simulink model "model"  (R2024b)
settings: Solver=ode1  StartTime=0.0  StopTime=10  FixedStep=0.0001  RelTol=1e-3
values from neighbouring files (symbols this model uses):
  a1 = c*a2    (= 810)    [init.m]
  a2 = c*a3    (= 270)    [init.m]
  a3 = c*a4    (= 90)    [init.m]
  a4 = c*10    (= 30)    [init.m]
  c1 = 50    [init.m]
  c2 = 1    [init.m]
  d = 100    [init.m]
  dis_gain = 30    [init.m]
  epsilon = 1    [init.m]
  i = 20    [init.m]
  k = 5    [init.m]
  mu = 0.9    [init.m]
  p = 400    [init.m]
  phi_frist = 0    [init.m]
  psi_frist = 0    [init.m]
  tau_p_max = 3000000    [init.m]
  theta_frist = 0    [init.m]
  umax = pi/2 - 0.01    (= 1.56079632679)    [init.m]
  w = wo    (= 50)    [init.m]
  wo = 50    [init.m]
  x_frist = 0    [init.m]
  y_frist = 0    [init.m]
  z_frist = 0    [init.m]
libraries: fod x36, slpidlib x6, simulink x1
(part 1 of 4)
settings Model: Creator=qians  LastModifiedBy=qians

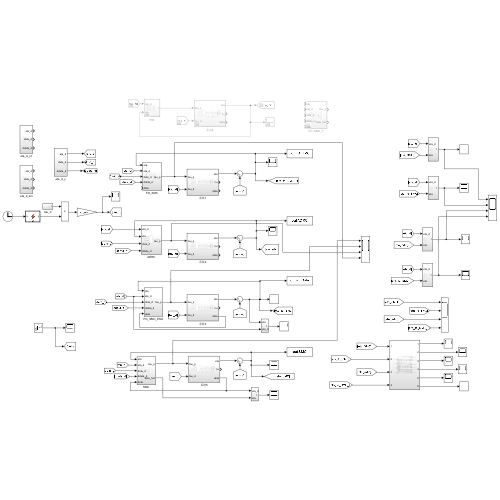
[thumbnail: Simulink's stored preview of the top-level diagram]
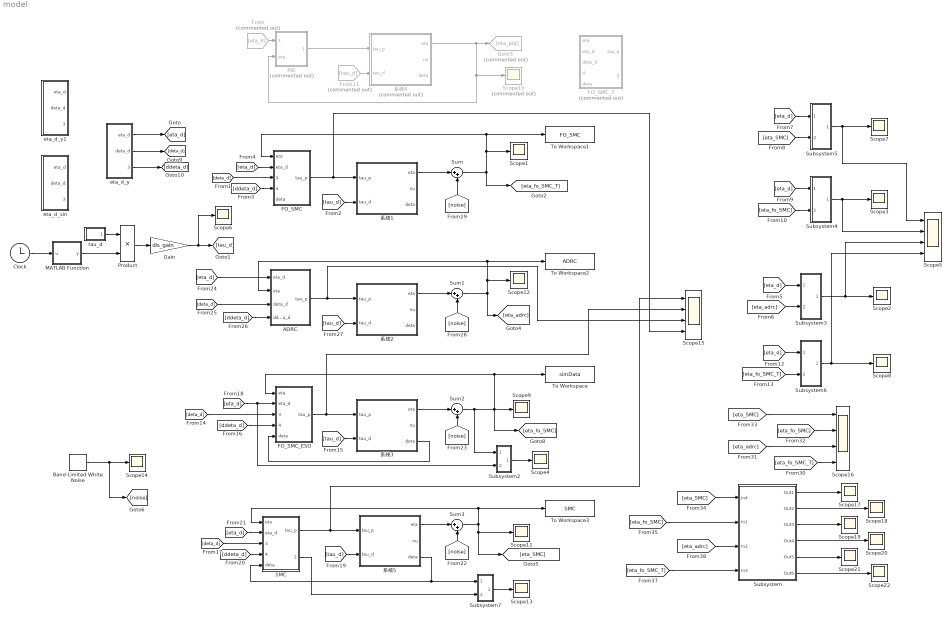
== system model ==
  ADRC : Subsystem
  Band-Limited White Noise : simulink/Sources/Band-Limited White Noise  Cov=[0.00001]  Ts=0.001  seed=[23341]
  Clock : Clock
  FO_SMC : Subsystem
  FO_SMC_ESO : Subsystem
  FO_SMC_T : Subsystem  Commented=on
  From : From  Commented=on  GotoTag=eta_d
  From11 : From  Commented=on  GotoTag=tau_d
  Gain : Gain  Gain=dis_gain
  Goto3 : Goto  Commented=on  GotoTag=eta_pid
  MATLAB Function : MATLAB Function  TreatAsAtomicUnit=on
  PID : Subsystem  Commented=on
  Product : Product
  SMC : Subsystem
  Scope{1..4,6..9,11..14,17..22} (18 alike) : Scope
  Scope10 : Scope  Commented=on
  Scope15 : Scope  NumInputPorts=4
  Scope16 : Scope  NumInputPorts=4
  Scope5 : Scope  NumInputPorts=4
  Subsystem : Subsystem
  Subsystem2 : Subsystem
  Subsystem3 : Subsystem
  Subsystem4 : Subsystem
  Subsystem5 : Subsystem
  Subsystem6 : Subsystem
  Subsystem7 : Subsystem
  Sum{,1..3} (4 alike) : Sum  Inputs=|++
  To Workspace : ToWorkspace  VariableName=simData  SaveFormat=Structure With Time  SampleTime=-1
  To Workspace1 : ToWorkspace  VariableName=FO_SMC  SaveFormat=Structure With Time  SampleTime=-1
  To Workspace2 : ToWorkspace  VariableName=ADRC  SaveFormat=Structure With Time  SampleTime=-1
  To Workspace3 : ToWorkspace  VariableName=SMC  SaveFormat=Structure With Time  SampleTime=-1
  eta_d_sin : Subsystem
  eta_d_y : Subsystem
  eta_d_y1 : Subsystem
  tau_d : Subsystem
  系统1 : Subsystem
  系统2 : Subsystem
  系统3 : Subsystem
  系统4 : Subsystem  Commented=on
  系统5 : Subsystem
  wires:
  Sum2/1 -> Subsystem2/1(eta), FO_SMC_ESO/1(eta), To Workspace/1, Scope9/1, [eta_fo_SMC]
  eta_d_y/2(deta_d) -> [deta_d]
  eta_d_y/1(eta_d) -> [eta_d]
  [deta_d] -> FO_SMC_ESO/3(deta_d)
  [ddeta_d] -> FO_SMC_ESO/4(ddeta_d)
  系统3/3(deta) -> FO_SMC_ESO/5(deta)
  [eta_d] -> FO_SMC_ESO/2(eta_d), Subsystem2/2(eta_d)
  eta_d_y/3(ddeta_d) -> [ddeta_d]
  FO_SMC_ESO/1(tau_p) -> 系统3/1(tau_p), Scope15/2
  [tau_d] -> 系统3/2(tau_d)
  Subsystem2/1(Out1) -> Scope4/1
  [ddeta_d] -> FO_SMC/4(ddeta_d)
  [tau_d] -> 系统1/2(tau_d)
  FO_SMC/1(tau_p) -> 系统1/1(tau_p), Scope15/4
  [eta_d] -> FO_SMC/2(eta_d)
  Sum/1 -> To Workspace1/1, FO_SMC/1(eta), Scope1/1, [eta_fo_SMC_T]
  [deta_d] -> FO_SMC/3(deta_d)
  [eta_SMC] -> Subsystem5/2(eta)
  [eta_fo_SMC_T] -> Subsystem6/2(eta)
  [eta_d] -> Subsystem3/1(eta_d)
  [eta_adrc] -> Subsystem3/2(eta)
  [eta_d] -> Subsystem5/1(eta_d)
  [eta_d] -> Subsystem4/1(eta_d)
  Subsystem3/1(Out1) -> Scope5/3, Scope2/1
  Subsystem5/1(Out1) -> Scope5/1, Scope7/1
  [eta_d] -> Subsystem6/1(eta_d)
  [eta_fo_SMC] -> Subsystem4/2(eta)
  Subsystem6/1(Out1) -> Scope5/4, Scope8/1
  Subsystem4/1(Out1) -> Scope5/2, Scope3/1
  From11/1 -> 系统4/2(tau_d)
  From/1 -> PID/1(eta_d)
  PID/1(Out1) -> 系统4/1(tau_p)
  系统4/1(eta) -> Scope10/1, PID/2(eta), Goto3/1
  [ddeta_d] -> ADRC/4(ddeta_d)
  ADRC/1(tau_p) -> Scope15/3, 系统2/1(tau_p)
  [tau_d] -> 系统2/2(tau_d)
  Sum1/1 -> ADRC/2(eta), To Workspace2/1, Scope12/1, [eta_adrc]
  [deta_d] -> ADRC/3(deta_d)
  [eta_d] -> ADRC/1(eta_d)
  [ddeta_d] -> SMC/4(ddeta_d)
  [deta_d] -> SMC/3(deta_d)
  [eta_d] -> SMC/2(eta_d)
  SMC/1(tau_p) -> 系统5/1(tau_p), Scope15/1
  Sum3/1 -> Scope11/1, [eta_SMC], SMC/1(eta), To Workspace3/1
  系统5/3(deta) -> SMC/5(deta), Subsystem7/1(eta_d)
  Subsystem7/1(Out1) -> Scope13/1
  [tau_d] -> 系统5/2(tau_d)
  SMC/2(deta_hat) -> Subsystem7/2(eta)
  Gain/1 -> [tau_d], Scope6/1
  Band-Limited White Noise/1 -> [noise], Scope14/1
  系统1/1(eta) -> Sum/1
  系统2/1(eta) -> Sum1/1
  系统3/1(eta) -> Sum2/1
  系统5/1(eta) -> Sum3/1
  [noise] -> Sum1/2
  [noise] -> Sum/2
  tau_d/1(Out1) -> Product/1
  Product/1 -> Gain/1
  Clock/1 -> MATLAB Function/1(u)
  MATLAB Function/1(y) -> Product/2
  [eta_fo_SMC_T] -> Scope16/4
  [eta_adrc] -> Scope16/3
  [eta_fo_SMC] -> Scope16/2
  [eta_SMC] -> Scope16/1
  [eta_SMC] -> Subsystem/1(In4)
  [eta_fo_SMC] -> Subsystem/2(In1)
  [eta_adrc] -> Subsystem/3(In2)
  [eta_fo_SMC_T] -> Subsystem/4(In3)
  Subsystem/1(Out1) -> Scope17/1
  Subsystem/2(Out2) -> Scope18/1
  Subsystem/3(Out3) -> Scope19/1
  Subsystem/4(Out4) -> Scope20/1
  Subsystem/5(Out5) -> Scope21/1
  Subsystem/6(Out6) -> Scope22/1
  [noise] -> Sum2/2
  [noise] -> Sum3/2

== system model/ADRC ==
  eta_d : Inport
  eta : Inport  Port=2
  deta_d : Inport  Port=3
  ddeta_d : Inport  Port=4
  控制器 : Subsystem
  tau_p : Outport
  wires:
  ddeta_d/1 -> 控制器/4(ddr)
  deta_d/1 -> 控制器/3(dr)
  eta/1 -> 控制器/2(eta)
  eta_d/1 -> 控制器/1(r)
  控制器/1(tau_p) -> tau_p/1

== system model/FO_SMC ==
  eta : Inport
  eta_d : Inport  Port=2
  deta_d : Inport  Port=3
  ddeta_d : Inport  Port=4
  deta : Inport  Port=5
  Constant : Constant  Value=c1
  Constant1 : Constant  Value=c2
  Constant2 : Constant  Value=k
  Constant3 : Constant  Value=epsilon
  MATLAB Function : MATLAB Function  TreatAsAtomicUnit=on
  MATLAB Function1 : MATLAB Function  TreatAsAtomicUnit=on
  Subsystem : Subsystem
  Subsystem2 : Subsystem
  tau_p : Outport
  wires:
  MATLAB Function1/1(nu) -> MATLAB Function/6(nu)
  eta_d/1 -> Subsystem2/2(eta_d), MATLAB Function/2(eta_d)
  ddeta_d/1 -> MATLAB Function/5(ddeta_d)
  eta/1 -> Subsystem/1(y), MATLAB Function1/1(eta), Subsystem2/1(eta), MATLAB Function/1(eta)
  Subsystem2/1(Out1) -> MATLAB Function/7(D1)
  Subsystem2/2(Out2) -> MATLAB Function/8(D2)
  deta_d/1 -> MATLAB Function/4(deta_d)
  Subsystem/2(y1_hat) -> MATLAB Function/3(deta), MATLAB Function1/2(deta)
  Constant/1 -> MATLAB Function/9(c1)
  Constant1/1 -> MATLAB Function/10(c2)
  Constant2/1 -> MATLAB Function/11(k)
  Constant3/1 -> MATLAB Function/12(epsilon)
  MATLAB Function/1(tau_p) -> tau_p/1

== system model/FO_SMC_ESO ==
  eta : Inport
  eta_d : Inport  Port=2
  deta_d : Inport  Port=3
  ddeta_d : Inport  Port=4
  deta : Inport  Port=5
  LESO : Subsystem
  Levant微分器 : Subsystem
  MATLAB Function : MATLAB Function  TreatAsAtomicUnit=on
  Subsystem1 : Subsystem
  Subsystem2 : Subsystem
  Subsystem3 : Subsystem
  Sum1 : Sum  Inputs=|++
  tau_p : Outport
  wires:
  Sum1/1 -> MATLAB Function/2(u2), LESO/5(tau_c)
  LESO/1(tau_2) -> Sum1/1
  eta/1 -> Subsystem3/1(eta), Subsystem2/1(eta), LESO/1(eta), Levant微分器/1(y), Subsystem2/3(eta1), Subsystem3/2(eta1)
  Levant微分器/2(y1_hat) -> Subsystem2/2(deta), Subsystem3/5(deta), Subsystem2/4(deta1)
  Subsystem1/1(Out1) -> tau_p/1
  MATLAB Function/1(y) -> Subsystem1/1(y)
  Subsystem3/1(tau_3) -> Sum1/2
  eta_d/1 -> Subsystem3/6(eta_d)
  deta_d/1 -> Subsystem3/7(deta_d)
  ddeta_d/1 -> Subsystem3/8(ddeta_d)
  Subsystem2/3(J) -> Subsystem3/4(J), LESO/3(J)
  Subsystem2/2(M_eta) -> Subsystem3/3(M_eta), LESO/2(M_eta)
  Subsystem2/1(tau_1) -> MATLAB Function/1(u1)
  Subsystem2/4(J_inv) -> LESO/4(J_inv)
  LESO/2(h3) -> Subsystem3/9(h3)

== system model/FO_SMC_T ==
  eta : Inport
  eta_d : Inport  Port=2
  deta_d : Inport  Port=3
  ddeta_d : Inport  Port=4
  deta : Inport  Port=5
  Constant1 : Constant  Value=c1
  Constant2 : Constant  Value=k
  Constant3 : Constant  Value=epsilon
  Constant4 : Constant  Value=c2
  MATLAB Function : MATLAB Function  TreatAsAtomicUnit=on
  MATLAB Function1 : MATLAB Function  TreatAsAtomicUnit=on
  Subsystem : Subsystem
  Subsystem2 : Subsystem
  tau_p : Outport
  deta_hat : Outport  Port=2
  wires:
  MATLAB Function/1(tau_p) -> tau_p/1
  MATLAB Function1/1(nu) -> MATLAB Function/6(nu)
  eta_d/1 -> Subsystem2/2(eta_d), MATLAB Function/2(eta_d)
  ddeta_d/1 -> MATLAB Function/5(ddeta_d)
  Subsystem2/1(Out1) -> MATLAB Function/7(D1)
  Subsystem2/2(Out2) -> MATLAB Function/8(D2)
  deta_d/1 -> MATLAB Function/4(deta_d)
  Subsystem/2(y1_hat) -> MATLAB Function/3(deta), MATLAB Function1/2(deta), deta_hat/1
  eta/1 -> Subsystem/1(y), Subsystem2/1(eta), MATLAB Function1/1(eta)
  Subsystem/1(y_hat) -> MATLAB Function/1(eta)
  Constant2/1 -> MATLAB Function/9(k)
  Constant3/1 -> MATLAB Function/10(epsilon)
  Constant1/1 -> MATLAB Function/11(c1)
  Constant4/1 -> MATLAB Function/12(c2)

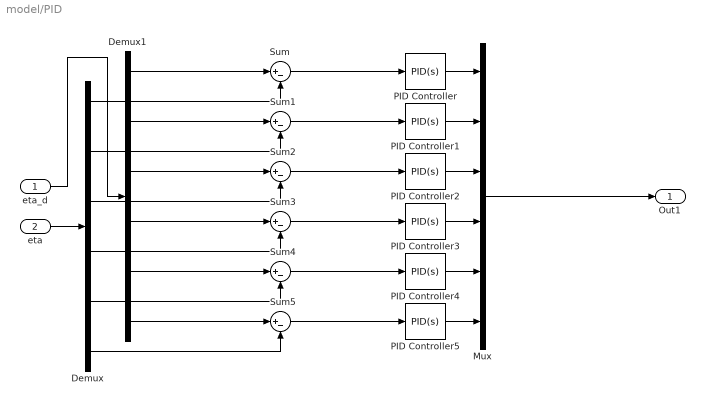
== system model/PID ==
  eta_d : Inport
  eta : Inport  Port=2
  Demux : Demux  Outputs=6
  Demux1 : Demux  Outputs=6
  Mux : Mux  Inputs=6
  PID Controller{,1..5} (6 alike) : slpidlib/PID Controller  Controller=PID  Form=Parallel  TimeDomain=Continuous-time  UseExternalTs=off  SampleTime=-1  IntegratorMethod=Forward Euler  FilterMethod=Forward Euler  ControllerParametersSource=internal  P=p  I=i  UseKiTs=off  D=d  UseExternalDerivativeSource=off  N=100  UseFilter=on  TunerSelectOption=Transfer Function Based (PID Tuner App)  InitialConditionSource=internal  InitialConditionForIntegrator=0  InitialConditionForFilter=0  DifferentiatorICPrevScaledInput=0  ExternalReset=none  TrackingMode=off  Kt=1  LimitOutput=off  SatLimitsSource=internal  UpperSaturationLimit=inf  LowerSaturationLimit=-inf  LinearizeAsGain=on  AntiWindupMode=none  Kb=1  LimitIntegrator=off  UpperIntegratorSaturationLimit=inf  LowerIntegratorSaturationLimit=-inf  POutMin=[]  POutMax=[]  IOutMin=[]  IOutMax=[]  DOutMin=[]  DOutMax=[]  NOutMin=[]  NOutMax=[]  SumOutMin=[]  SumOutMax=[]  SaturationOutMin=[]  SaturationOutMax=[]  PParamMin=[]  PParamMax=[]  IParamMin=[]  IParamMax=[]  DParamMin=[]  DParamMax=[]  NParamMin=[]  NParamMax=[]  KbParamMin=[]  KbParamMax=[]  KtParamMin=[]  KtParamMax=[]  KbOutMin=[]  KbOutMax=[]  KtOutMin=[]  KtOutMax=[]  IntegratorOutMin=[]  IntegratorOutMax=[]  FilterOutMin=[]  FilterOutMax=[]  SumI1OutMin=[]  SumI1OutMax=[]  SumI2OutMin=[]  SumI2OutMax=[]  SumI3OutMin=[]  SumI3OutMax=[]  SumI4OutMin=[]  SumI4OutMax=[]  SumDOutMin=[]  SumDOutMax=[]  DifferentiatorOutMin=[]  DifferentiatorOutMax=[]  FilterDiffOutCoefMin=[]  FilterDiffOutCoefMax=[]  ReciprocalOutMin=[]  ReciprocalOutMax=[]  SumDenOutMin=[]  SumDenOutMax=[]  SumNumOutMin=[]  SumNumOutMax=[]  DivideOutMin=[]  DivideOutMax=[]  UdiffTsProdOutMin=[]  UdiffTsProdOutMax=[]  NTsProdOutMin=[]  NTsProdOutMax=[]  UintegralTsProdOutMin=[]  UintegralTsProdOutMax=[]  UngainTsProdOutMin=[]  UngainTsProdOutMax=[]  ClampingZeroOutDataTypeStr=Inherit: Inherit via back propagation  ClampingZeroOutMin=[]  ClampingZeroOutMax=[]  FilterDenConstantOutDataTypeStr=Inherit: Inherit via back propagation  FilterDenConstantOutMin=[]  FilterDenConstantOutMax=[]  PCopyOutDataTypeStr=Inherit: Inherit via back propagation  PCopyOutMin=[]  PCopyOutMax=[]  NCopyOutDataTypeStr=Inherit: Inherit via back propagation  NCopyOutMin=[]  NCopyOutMax=[]  IntegratorContinuousStateAttributes=''  IntegratorStateMustResolveToSignalObject=off  IntegratorRTWStateStorageClass=Auto  FilterContinuousStateAttributes=''  FilterStateMustResolveToSignalObject=off  FilterRTWStateStorageClass=Auto  ParallelPVariant=InternalParameters  IdealPVariant=Disabled  IVariant=InternalParameters  DVariant=InternalParameters  IntegratorVariant=Continuous  SatVariant=Disabled  AWVariant=Passthrough  PCopyVariant=Disabled  TRVariant=Disabled  FdbkBlocksVariant=Forward  IdealPFdbkVariant=Disabled  SatFdbkVariant=Disabled  DerivativeFilterVariant=ContFilter  NVariant=InternalParameters  NCopyVariant=Disabled  FilterICVariant=InternalICsFilter  IntegratorICVariant=InternalICs  ExternalResetVariant=Disabled  TRSumVariant=Passthrough  SumFdbkVariant=Disabled  SumVariant=Sum_PID  TsampFilterVariant=InternalTs  TsampNgainVariant=Passthrough  TsampIntegralVariant=Disabled_SignalSpec  ExternalSaturationOutDataTypeStr=Inherit: Same as second input  DerivativeSourceVariant=ErrorSignal  PreIntVariant=InternalPreInt
  Sum{,1..5} (6 alike) : Sum  Inputs=|+-
  Out1 : Outport
  wires:
  PID Controller5/1 -> Mux/6
  PID Controller/1 -> Mux/1
  PID Controller4/1 -> Mux/5
  PID Controller2/1 -> Mux/3
  PID Controller1/1 -> Mux/2
  PID Controller3/1 -> Mux/4
  Mux/1 -> Out1/1
  eta/1 -> Demux/1
  Demux1/1 -> Sum/1
  Sum/1 -> PID Controller/1
  Demux/1 -> Sum/2
  Demux/2 -> Sum1/2
  Sum1/1 -> PID Controller1/1
  Demux1/2 -> Sum1/1
  Demux1/3 -> Sum2/1
  Sum2/1 -> PID Controller2/1
  Demux/3 -> Sum2/2
  Demux/4 -> Sum3/2
  Sum3/1 -> PID Controller3/1
  Demux1/4 -> Sum3/1
  Demux1/5 -> Sum4/1
  Sum4/1 -> PID Controller4/1
  Demux/5 -> Sum4/2
  Demux/6 -> Sum5/2
  Sum5/1 -> PID Controller5/1
  Demux1/6 -> Sum5/1
  eta_d/1 -> Demux1/1

== system model/SMC ==
  eta : Inport
  eta_d : Inport  Port=2
  deta_d : Inport  Port=3
  ddeta_d : Inport  Port=4
  deta : Inport  Port=5
  Constant : Constant  Value=c1
  Constant2 : Constant  Value=k
  Constant3 : Constant  Value=epsilon
  MATLAB Function : MATLAB Function  TreatAsAtomicUnit=on
  MATLAB Function1 : MATLAB Function  TreatAsAtomicUnit=on
  Subsystem : Subsystem
  tau_p : Outport
  deta_hat : Outport  Port=2
  wires:
  MATLAB Function/1(tau_p) -> tau_p/1
  MATLAB Function1/1(nu) -> MATLAB Function/6(nu)
  eta_d/1 -> MATLAB Function/2(eta_d)
  ddeta_d/1 -> MATLAB Function/5(ddeta_d)
  eta/1 -> MATLAB Function/1(eta), MATLAB Function1/1(eta), Subsystem/1(y)
  deta_d/1 -> MATLAB Function/4(deta_d)
  Subsystem/2(y1_hat) -> deta_hat/1, MATLAB Function/3(deta), MATLAB Function1/2(deta)
  Constant/1 -> MATLAB Function/7(c1)
  Constant2/1 -> MATLAB Function/8(k)
  Constant3/1 -> MATLAB Function/9(epsilon)

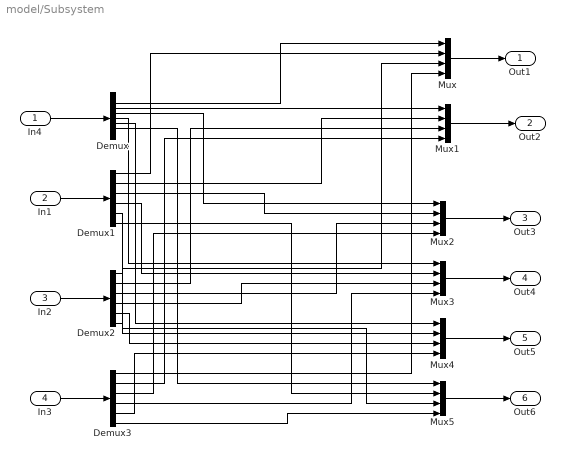
== system model/Subsystem ==
  In4 : Inport
  In1 : Inport  Port=2
  In2 : Inport  Port=3
  In3 : Inport  Port=4
  Demux{,1..3} (4 alike) : Demux  Outputs=6
  Mux{,1..5} (6 alike) : Mux
  Out1 : Outport
  Out2 : Outport  Port=2
  Out3 : Outport  Port=3
  Out4 : Outport  Port=4
  Out5 : Outport  Port=5
  Out6 : Outport  Port=6
  wires:
  Demux/1 -> Mux/1
  In4/1 -> Demux/1
  Mux/1 -> Out1/1
  In1/1 -> Demux1/1
  Demux1/1 -> Mux/2
  Demux/2 -> Mux1/1
  Demux1/2 -> Mux1/2
  Mux1/1 -> Out2/1
  Mux2/1 -> Out3/1
  Demux1/3 -> Mux2/2
  Demux/3 -> Mux2/1
  Demux/4 -> Mux3/1
  Demux1/4 -> Mux3/2
  Mux3/1 -> Out4/1
  Mux4/1 -> Out5/1
  Demux1/5 -> Mux4/2
  Demux/5 -> Mux4/1
  Demux/6 -> Mux5/1
  Demux1/6 -> Mux5/2
  Mux5/1 -> Out6/1
  In2/1 -> Demux2/1
  In3/1 -> Demux3/1
  Demux2/1 -> Mux/3
  Demux2/2 -> Mux1/3
  Demux2/3 -> Mux2/3
  Demux2/4 -> Mux3/3
  Demux2/5 -> Mux4/3
  Demux2/6 -> Mux5/3
  Demux3/1 -> Mux/4
  Demux3/2 -> Mux1/4
  Demux3/3 -> Mux2/4
  Demux3/4 -> Mux3/4
  Demux3/5 -> Mux4/4
  Demux3/6 -> Mux5/4

== system model/Subsystem2 ==
  eta : Inport
  eta_d : Inport  Port=2
  Demux : Demux  Outputs=6
  Demux1 : Demux  Outputs=6
  Mux : Mux  Inputs=6
  Sum{,1..5} (6 alike) : Sum  Inputs=|+-
  Out1 : Outport
  wires:
  eta_d/1 -> Demux1/1
  Demux1/6 -> Sum5/1
  Demux/6 -> Sum5/2
  Demux/5 -> Sum4/2
  Demux1/5 -> Sum4/1
  Demux1/4 -> Sum3/1
  Demux/4 -> Sum3/2
  Demux/3 -> Sum2/2
  Demux1/3 -> Sum2/1
  Demux1/2 -> Sum1/1
  Demux/2 -> Sum1/2
  Demux/1 -> Sum/2
  Demux1/1 -> Sum/1
  eta/1 -> Demux/1
  Mux/1 -> Out1/1
  Sum3/1 -> Mux/4
  Sum1/1 -> Mux/2
  Sum2/1 -> Mux/3
  Sum4/1 -> Mux/5
  Sum/1 -> Mux/1
  Sum5/1 -> Mux/6

== system model/Subsystem3 ==
  eta_d : Inport
  eta : Inport  Port=2
  Demux : Demux  Outputs=6
  Demux1 : Demux  Outputs=6
  Mux : Mux  Inputs=6
  Sum{,1..5} (6 alike) : Sum  Inputs=|+-
  Out1 : Outport
  wires:
  eta_d/1 -> Demux1/1
  Demux1/6 -> Sum5/1
  Demux/6 -> Sum5/2
  Demux/5 -> Sum4/2
  Demux1/5 -> Sum4/1
  Demux1/4 -> Sum3/1
  Demux/4 -> Sum3/2
  Demux/3 -> Sum2/2
  Demux1/3 -> Sum2/1
  Demux1/2 -> Sum1/1
  Demux/2 -> Sum1/2
  Demux/1 -> Sum/2
  Demux1/1 -> Sum/1
  eta/1 -> Demux/1
  Mux/1 -> Out1/1
  Sum3/1 -> Mux/4
  Sum1/1 -> Mux/2
  Sum2/1 -> Mux/3
  Sum4/1 -> Mux/5
  Sum/1 -> Mux/1
  Sum5/1 -> Mux/6

== system model/Subsystem4 ==
  eta_d : Inport
  eta : Inport  Port=2
  Demux : Demux  Outputs=6
  Demux1 : Demux  Outputs=6
  Mux : Mux  Inputs=6
  Sum{,1..5} (6 alike) : Sum  Inputs=|+-
  Out1 : Outport
  wires:
  Sum5/1 -> Mux/6
  Sum/1 -> Mux/1
  Sum4/1 -> Mux/5
  Sum2/1 -> Mux/3
  Sum1/1 -> Mux/2
  Sum3/1 -> Mux/4
  Mux/1 -> Out1/1
  eta/1 -> Demux/1
  Demux1/1 -> Sum/1
  Demux/1 -> Sum/2
  Demux/2 -> Sum1/2
  Demux1/2 -> Sum1/1
  Demux1/3 -> Sum2/1
  Demux/3 -> Sum2/2
  Demux/4 -> Sum3/2
  Demux1/4 -> Sum3/1
  Demux1/5 -> Sum4/1
  Demux/5 -> Sum4/2
  Demux/6 -> Sum5/2
  Demux1/6 -> Sum5/1
  eta_d/1 -> Demux1/1

== system model/Subsystem5 ==
  eta_d : Inport
  eta : Inport  Port=2
  Demux : Demux  Outputs=6
  Demux1 : Demux  Outputs=6
  Mux : Mux  Inputs=6
  Sum{,1..5} (6 alike) : Sum  Inputs=|+-
  Out1 : Outport
  wires:
  eta_d/1 -> Demux1/1
  Demux1/6 -> Sum5/1
  Demux/6 -> Sum5/2
  Demux/5 -> Sum4/2
  Demux1/5 -> Sum4/1
  Demux1/4 -> Sum3/1
  Demux/4 -> Sum3/2
  Demux/3 -> Sum2/2
  Demux1/3 -> Sum2/1
  Demux1/2 -> Sum1/1
  Demux/2 -> Sum1/2
  Demux/1 -> Sum/2
  Demux1/1 -> Sum/1
  eta/1 -> Demux/1
  Mux/1 -> Out1/1
  Sum3/1 -> Mux/4
  Sum1/1 -> Mux/2
  Sum2/1 -> Mux/3
  Sum4/1 -> Mux/5
  Sum/1 -> Mux/1
  Sum5/1 -> Mux/6

== system model/Subsystem6 ==
  eta_d : Inport
  eta : Inport  Port=2
  Demux : Demux  Outputs=6
  Demux1 : Demux  Outputs=6
  Mux : Mux  Inputs=6
  Sum{,1..5} (6 alike) : Sum  Inputs=|+-
  Out1 : Outport
  wires:
  Sum5/1 -> Mux/6
  Sum/1 -> Mux/1
  Sum4/1 -> Mux/5
  Sum2/1 -> Mux/3
  Sum1/1 -> Mux/2
  Sum3/1 -> Mux/4
  Mux/1 -> Out1/1
  eta/1 -> Demux/1
  Demux1/1 -> Sum/1
  Demux/1 -> Sum/2
  Demux/2 -> Sum1/2
  Demux1/2 -> Sum1/1
  Demux1/3 -> Sum2/1
  Demux/3 -> Sum2/2
  Demux/4 -> Sum3/2
  Demux1/4 -> Sum3/1
  Demux1/5 -> Sum4/1
  Demux/5 -> Sum4/2
  Demux/6 -> Sum5/2
  Demux1/6 -> Sum5/1
  eta_d/1 -> Demux1/1

== system model/Subsystem7 ==
  eta_d : Inport
  eta : Inport  Port=2
  Demux : Demux  Outputs=6
  Demux1 : Demux  Outputs=6
  Mux : Mux  Inputs=6
  Sum{,1..5} (6 alike) : Sum  Inputs=|+-
  Out1 : Outport
  wires:
  eta_d/1 -> Demux1/1
  Demux1/6 -> Sum5/1
  Demux/6 -> Sum5/2
  Demux/5 -> Sum4/2
  Demux1/5 -> Sum4/1
  Demux1/4 -> Sum3/1
  Demux/4 -> Sum3/2
  Demux/3 -> Sum2/2
  Demux1/3 -> Sum2/1
  Demux1/2 -> Sum1/1
  Demux/2 -> Sum1/2
  Demux/1 -> Sum/2
  Demux1/1 -> Sum/1
  eta/1 -> Demux/1
  Mux/1 -> Out1/1
  Sum3/1 -> Mux/4
  Sum1/1 -> Mux/2
  Sum2/1 -> Mux/3
  Sum4/1 -> Mux/5
  Sum/1 -> Mux/1
  Sum5/1 -> Mux/6

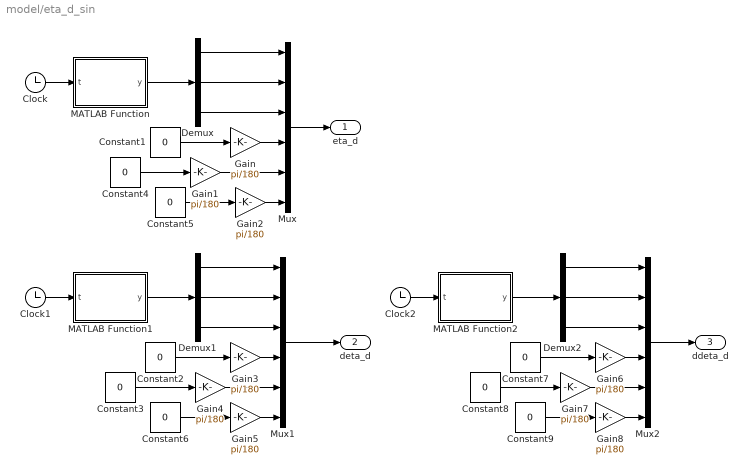
== system model/eta_d_sin ==
  Clock : Clock
  Clock1 : Clock
  Clock2 : Clock
  Constant{1..9} (9 alike) : Constant  Value=0
  Demux : Demux  Outputs=3
  Demux1 : Demux  Outputs=3
  Demux2 : Demux  Outputs=3
  Gain{,1..8} (9 alike) : Gain  Gain=pi/180
  MATLAB Function : MATLAB Function  TreatAsAtomicUnit=on
  MATLAB Function1 : MATLAB Function  TreatAsAtomicUnit=on
  MATLAB Function2 : MATLAB Function  TreatAsAtomicUnit=on
  Mux : Mux  Inputs=6
  Mux1 : Mux  Inputs=6
  Mux2 : Mux  Inputs=6
  eta_d : Outport
  deta_d : Outport  Port=2
  ddeta_d : Outport  Port=3
  wires:
  Gain2/1 -> Mux/6
  Demux/1 -> Mux/1
  Gain/1 -> Mux/4
  Constant4/1 -> Gain1/1
  Mux/1 -> eta_d/1
  Demux/3 -> Mux/3
  Demux/2 -> Mux/2
  Constant5/1 -> Gain2/1
  Gain1/1 -> Mux/5
  Constant1/1 -> Gain/1
  Clock/1 -> MATLAB Function/1(t)
  MATLAB Function/1(y) -> Demux/1
  MATLAB Function1/1(y) -> Demux1/1
  Clock1/1 -> MATLAB Function1/1(t)
  Constant2/1 -> Gain3/1
  Gain4/1 -> Mux1/5
  Constant6/1 -> Gain5/1
  Demux1/2 -> Mux1/2
  Demux1/3 -> Mux1/3
  Mux1/1 -> deta_d/1
  Constant3/1 -> Gain4/1
  Gain3/1 -> Mux1/4
  Demux1/1 -> Mux1/1
  Gain5/1 -> Mux1/6
  Gain8/1 -> Mux2/6
  Demux2/1 -> Mux2/1
  Gain6/1 -> Mux2/4
  Constant8/1 -> Gain7/1
  Mux2/1 -> ddeta_d/1
  Demux2/3 -> Mux2/3
  Demux2/2 -> Mux2/2
  Constant9/1 -> Gain8/1
  Gain7/1 -> Mux2/5
  Constant7/1 -> Gain6/1
  Clock2/1 -> MATLAB Function2/1(t)
  MATLAB Function2/1(y) -> Demux2/1

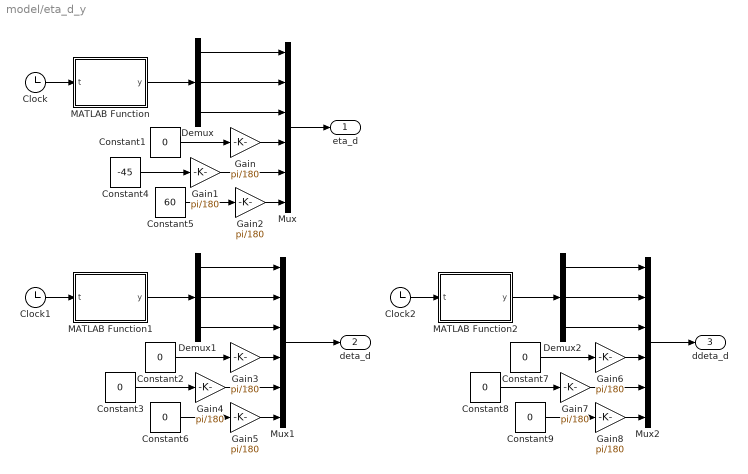
== system model/eta_d_y ==
  Clock : Clock
  Clock1 : Clock
  Clock2 : Clock
  Constant{1..3,6..9} (7 alike) : Constant  Value=0
  Constant4 : Constant  Value=-45
  Constant5 : Constant  Value=60
  Demux : Demux  Outputs=3
  Demux1 : Demux  Outputs=3
  Demux2 : Demux  Outputs=3
  Gain{,1..8} (9 alike) : Gain  Gain=pi/180
  MATLAB Function : MATLAB Function  TreatAsAtomicUnit=on
  MATLAB Function1 : MATLAB Function  TreatAsAtomicUnit=on
  MATLAB Function2 : MATLAB Function  TreatAsAtomicUnit=on
  Mux : Mux  Inputs=6
  Mux1 : Mux  Inputs=6
  Mux2 : Mux  Inputs=6
  eta_d : Outport
  deta_d : Outport  Port=2
  ddeta_d : Outport  Port=3
  wires:
  Gain2/1 -> Mux/6
  Demux/1 -> Mux/1
  Gain/1 -> Mux/4
  Constant4/1 -> Gain1/1
  Mux/1 -> eta_d/1
  Demux/3 -> Mux/3
  Demux/2 -> Mux/2
  Constant5/1 -> Gain2/1
  Gain1/1 -> Mux/5
  Constant1/1 -> Gain/1
  Clock/1 -> MATLAB Function/1(t)
  MATLAB Function/1(y) -> Demux/1
  MATLAB Function1/1(y) -> Demux1/1
  Clock1/1 -> MATLAB Function1/1(t)
  Constant2/1 -> Gain3/1
  Gain4/1 -> Mux1/5
  Constant6/1 -> Gain5/1
  Demux1/2 -> Mux1/2
  Demux1/3 -> Mux1/3
  Mux1/1 -> deta_d/1
  Constant3/1 -> Gain4/1
  Gain3/1 -> Mux1/4
  Demux1/1 -> Mux1/1
  Gain5/1 -> Mux1/6
  Gain8/1 -> Mux2/6
  Demux2/1 -> Mux2/1
  Gain6/1 -> Mux2/4
  Constant8/1 -> Gain7/1
  Mux2/1 -> ddeta_d/1
  Demux2/3 -> Mux2/3
  Demux2/2 -> Mux2/2
  Constant9/1 -> Gain8/1
  Gain7/1 -> Mux2/5
  Constant7/1 -> Gain6/1
  Clock2/1 -> MATLAB Function2/1(t)
  MATLAB Function2/1(y) -> Demux2/1

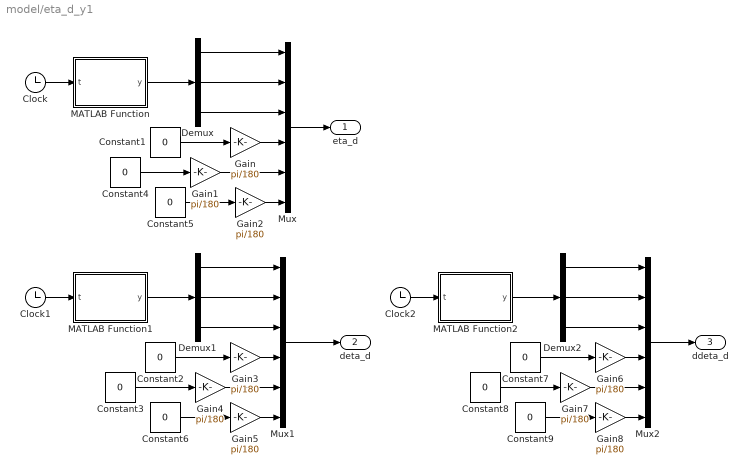
== system model/eta_d_y1 ==
  Clock : Clock
  Clock1 : Clock
  Clock2 : Clock
  Constant{1..9} (9 alike) : Constant  Value=0
  Demux : Demux  Outputs=3
  Demux1 : Demux  Outputs=3
  Demux2 : Demux  Outputs=3
  Gain{,1..8} (9 alike) : Gain  Gain=pi/180
  MATLAB Function : MATLAB Function  TreatAsAtomicUnit=on
  MATLAB Function1 : MATLAB Function  TreatAsAtomicUnit=on
  MATLAB Function2 : MATLAB Function  TreatAsAtomicUnit=on
  Mux : Mux  Inputs=6
  Mux1 : Mux  Inputs=6
  Mux2 : Mux  Inputs=6
  eta_d : Outport
  deta_d : Outport  Port=2
  ddeta_d : Outport  Port=3
  wires:
  MATLAB Function2/1(y) -> Demux2/1
  Clock2/1 -> MATLAB Function2/1(t)
  Constant7/1 -> Gain6/1
  Gain7/1 -> Mux2/5
  Constant9/1 -> Gain8/1
  Demux2/2 -> Mux2/2
  Demux2/3 -> Mux2/3
  Mux2/1 -> ddeta_d/1
  Constant8/1 -> Gain7/1
  Gain6/1 -> Mux2/4
  Demux2/1 -> Mux2/1
  Gain8/1 -> Mux2/6
  Gain5/1 -> Mux1/6
  Demux1/1 -> Mux1/1
  Gain3/1 -> Mux1/4
  Constant3/1 -> Gain4/1
  Mux1/1 -> deta_d/1
  Demux1/3 -> Mux1/3
  Demux1/2 -> Mux1/2
  Constant6/1 -> Gain5/1
  Gain4/1 -> Mux1/5
  Constant2/1 -> Gain3/1
  Clock1/1 -> MATLAB Function1/1(t)
  MATLAB Function1/1(y) -> Demux1/1
  MATLAB Function/1(y) -> Demux/1
  Clock/1 -> MATLAB Function/1(t)
  Constant1/1 -> Gain/1
  Gain1/1 -> Mux/5
  Constant5/1 -> Gain2/1
  Demux/2 -> Mux/2
  Demux/3 -> Mux/3
  Mux/1 -> eta_d/1
  Constant4/1 -> Gain1/1
  Gain/1 -> Mux/4
  Demux/1 -> Mux/1
  Gain2/1 -> Mux/6

== system model/tau_d ==
  Clock : Clock
  Clock1 : Clock
  Demux : Demux  Outputs=3
  Demux1 : Demux  Outputs=3
  Gain2 : Gain  Gain=pi/180
  MATLAB Function : MATLAB Function  TreatAsAtomicUnit=on
  MATLAB Function1 : MATLAB Function  TreatAsAtomicUnit=on
  Mux1 : Mux  Inputs=6
  Out1 : Outport
  wires:
  Mux1/1 -> Out1/1
  Clock/1 -> MATLAB Function/1(t)
  Demux/3 -> Mux1/3
  Demux/2 -> Mux1/2
  Demux/1 -> Mux1/1
  Demux1/1 -> Mux1/4
  Demux1/3 -> Mux1/6
  MATLAB Function/1(y) -> Demux/1
  Clock1/1 -> MATLAB Function1/1(t)
  MATLAB Function1/1(y) -> Gain2/1
  Gain2/1 -> Demux1/1
  Demux1/2 -> Mux1/5

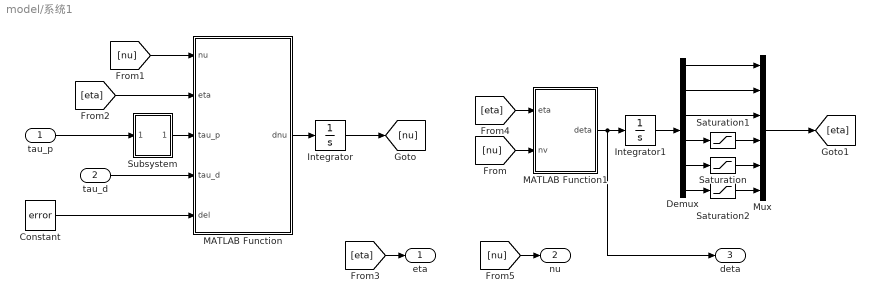
== system model/系统1 ==
  tau_p : Inport
  tau_d : Inport  Port=2
  Constant : Constant  Value=error
  Demux : Demux  Outputs=6
  Integrator : Integrator  InitialCondition=[0;0;0;0;0;0]
  Integrator1 : Integrator  InitialCondition=[x_frist;y_frist;z_frist;phi_frist;theta_frist;psi_frist]
  MATLAB Function : MATLAB Function  TreatAsAtomicUnit=on
  MATLAB Function1 : MATLAB Function  TreatAsAtomicUnit=on
  Mux : Mux  Inputs=6
  Saturation : Saturate  UpperLimit=umax  LowerLimit=-umax
  Saturation1 : Saturate  UpperLimit=umax  LowerLimit=-umax
  Saturation2 : Saturate  UpperLimit=umax  LowerLimit=-umax
  Subsystem : Subsystem
  eta : Outport
  nu : Outport  Port=2
  deta : Outport  Port=3
  wires:
  Subsystem/1(Out1) -> MATLAB Function/3(tau_p)
  Saturation/1 -> Mux/5
  Mux/1 -> [eta]
  Demux/6 -> Saturation2/1
  Demux/5 -> Saturation/1
  Demux/4 -> Saturation1/1
  Demux/3 -> Mux/3
  Demux/2 -> Mux/2
  Demux/1 -> Mux/1
  tau_d/1 -> MATLAB Function/4(tau_d)
  MATLAB Function1/1(deta) -> deta/1, Integrator1/1
  Integrator/1 -> [nu]
  Integrator1/1 -> Demux/1
  tau_p/1 -> Subsystem/1(In1)
  MATLAB Function/1(dnu) -> Integrator/1
  Saturation1/1 -> Mux/4
  [nu] -> MATLAB Function1/2(nv)
  [nu] -> MATLAB Function/1(nu)
  [eta] -> MATLAB Function/2(eta)
  [eta] -> eta/1
  [eta] -> MATLAB Function1/1(eta)
  [nu] -> nu/1
  Saturation2/1 -> Mux/6
  Constant/1 -> MATLAB Function/5(del)

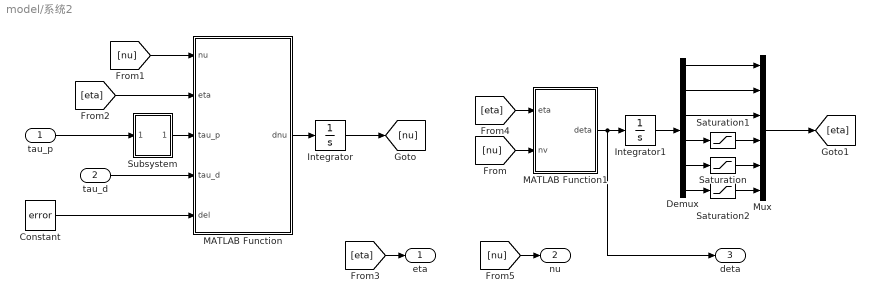
== system model/系统2 ==
  tau_p : Inport
  tau_d : Inport  Port=2
  Constant : Constant  Value=error
  Demux : Demux  Outputs=6
  Integrator : Integrator  InitialCondition=[0;0;0;0;0;0]
  Integrator1 : Integrator  InitialCondition=[x_frist;y_frist;z_frist;phi_frist;theta_frist;psi_frist]
  MATLAB Function : MATLAB Function  TreatAsAtomicUnit=on
  MATLAB Function1 : MATLAB Function  TreatAsAtomicUnit=on
  Mux : Mux  Inputs=6
  Saturation : Saturate  UpperLimit=umax  LowerLimit=-umax
  Saturation1 : Saturate  UpperLimit=umax  LowerLimit=-umax
  Saturation2 : Saturate  UpperLimit=umax  LowerLimit=-umax
  Subsystem : Subsystem
  eta : Outport
  nu : Outport  Port=2
  deta : Outport  Port=3
  wires:
  Constant/1 -> MATLAB Function/5(del)
  Saturation2/1 -> Mux/6
  [nu] -> nu/1
  [eta] -> MATLAB Function1/1(eta)
  [eta] -> eta/1
  [eta] -> MATLAB Function/2(eta)
  [nu] -> MATLAB Function/1(nu)
  [nu] -> MATLAB Function1/2(nv)
  Saturation1/1 -> Mux/4
  MATLAB Function/1(dnu) -> Integrator/1
  tau_p/1 -> Subsystem/1(In1)
  Integrator1/1 -> Demux/1
  Integrator/1 -> [nu]
  MATLAB Function1/1(deta) -> Integrator1/1, deta/1
  tau_d/1 -> MATLAB Function/4(tau_d)
  Demux/1 -> Mux/1
  Demux/2 -> Mux/2
  Demux/3 -> Mux/3
  Demux/4 -> Saturation1/1
  Demux/5 -> Saturation/1
  Demux/6 -> Saturation2/1
  Mux/1 -> [eta]
  Saturation/1 -> Mux/5
  Subsystem/1(Out1) -> MATLAB Function/3(tau_p)

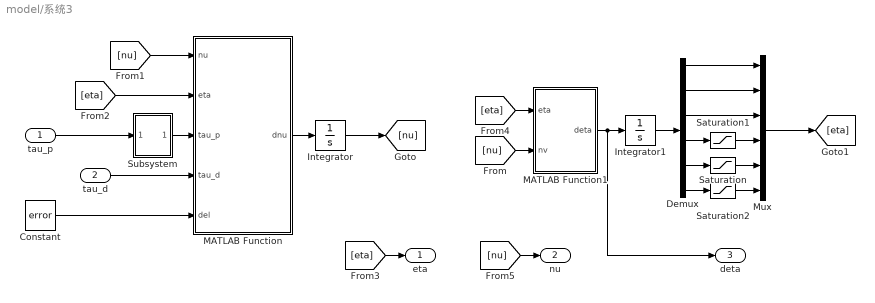
== system model/系统3 ==
  tau_p : Inport
  tau_d : Inport  Port=2
  Constant : Constant  Value=error
  Demux : Demux  Outputs=6
  Integrator : Integrator  InitialCondition=[0;0;0;0;0;0]
  Integrator1 : Integrator  InitialCondition=[x_frist;y_frist;z_frist;phi_frist;theta_frist;psi_frist]
  MATLAB Function : MATLAB Function  TreatAsAtomicUnit=on
  MATLAB Function1 : MATLAB Function  TreatAsAtomicUnit=on
  Mux : Mux  Inputs=6
  Saturation : Saturate  UpperLimit=umax  LowerLimit=-umax
  Saturation1 : Saturate  UpperLimit=umax  LowerLimit=-umax
  Saturation2 : Saturate  UpperLimit=umax  LowerLimit=-umax
  Subsystem : Subsystem
  eta : Outport
  nu : Outport  Port=2
  deta : Outport  Port=3
  wires:
  Subsystem/1(Out1) -> MATLAB Function/3(tau_p)
  Saturation/1 -> Mux/5
  Mux/1 -> [eta]
  Demux/6 -> Saturation2/1
  Demux/5 -> Saturation/1
  Demux/4 -> Saturation1/1
  Demux/3 -> Mux/3
  Demux/2 -> Mux/2
  Demux/1 -> Mux/1
  tau_d/1 -> MATLAB Function/4(tau_d)
  MATLAB Function1/1(deta) -> deta/1, Integrator1/1
  Integrator/1 -> [nu]
  Integrator1/1 -> Demux/1
  tau_p/1 -> Subsystem/1(In1)
  MATLAB Function/1(dnu) -> Integrator/1
  Saturation1/1 -> Mux/4
  [nu] -> MATLAB Function1/2(nv)
  [nu] -> MATLAB Function/1(nu)
  [eta] -> MATLAB Function/2(eta)
  [eta] -> eta/1
  [eta] -> MATLAB Function1/1(eta)
  [nu] -> nu/1
  Saturation2/1 -> Mux/6
  Constant/1 -> MATLAB Function/5(del)

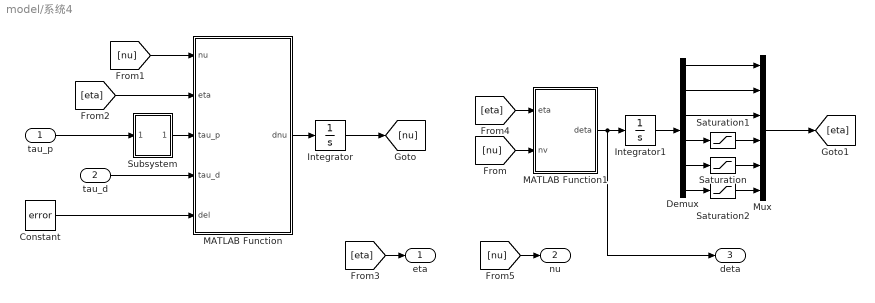
== system model/系统4 ==
  tau_p : Inport
  tau_d : Inport  Port=2
  Constant : Constant  Value=error
  Demux : Demux  Outputs=6
  Integrator : Integrator  InitialCondition=[0;0;0;0;0;0]
  Integrator1 : Integrator  InitialCondition=[1;1;0;0;0;0]
  MATLAB Function : MATLAB Function  TreatAsAtomicUnit=on
  MATLAB Function1 : MATLAB Function  TreatAsAtomicUnit=on
  Mux : Mux  Inputs=6
  Saturation : Saturate  UpperLimit=umax  LowerLimit=-umax
  Saturation1 : Saturate  UpperLimit=umax  LowerLimit=-umax
  Saturation2 : Saturate  UpperLimit=umax  LowerLimit=-umax
  Subsystem : Subsystem
  eta : Outport
  nu : Outport  Port=2
  deta : Outport  Port=3
  wires:
  Constant/1 -> MATLAB Function/5(del)
  Saturation2/1 -> Mux/6
  [nu] -> nu/1
  [eta] -> MATLAB Function1/1(eta)
  [eta] -> eta/1
  [eta] -> MATLAB Function/2(eta)
  [nu] -> MATLAB Function/1(nu)
  [nu] -> MATLAB Function1/2(nv)
  Saturation1/1 -> Mux/4
  MATLAB Function/1(dnu) -> Integrator/1
  tau_p/1 -> Subsystem/1(In1)
  Integrator1/1 -> Demux/1
  Integrator/1 -> [nu]
  MATLAB Function1/1(deta) -> Integrator1/1, deta/1
  tau_d/1 -> MATLAB Function/4(tau_d)
  Demux/1 -> Mux/1
  Demux/2 -> Mux/2
  Demux/3 -> Mux/3
  Demux/4 -> Saturation1/1
  Demux/5 -> Saturation/1
  Demux/6 -> Saturation2/1
  Mux/1 -> [eta]
  Saturation/1 -> Mux/5
  Subsystem/1(Out1) -> MATLAB Function/3(tau_p)

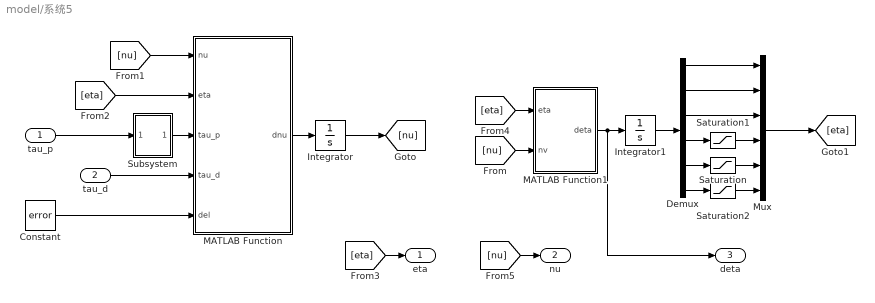
== system model/系统5 ==
  tau_p : Inport
  tau_d : Inport  Port=2
  Constant : Constant  Value=error
  Demux : Demux  Outputs=6
  Integrator : Integrator  InitialCondition=[0;0;0;0;0;0]
  Integrator1 : Integrator  InitialCondition=[x_frist;y_frist;z_frist;phi_frist;theta_frist;psi_frist]
  MATLAB Function : MATLAB Function  TreatAsAtomicUnit=on
  MATLAB Function1 : MATLAB Function  TreatAsAtomicUnit=on
  Mux : Mux  Inputs=6
  Saturation : Saturate  UpperLimit=umax  LowerLimit=-umax
  Saturation1 : Saturate  UpperLimit=umax  LowerLimit=-umax
  Saturation2 : Saturate  UpperLimit=umax  LowerLimit=-umax
  Subsystem : Subsystem
  eta : Outport
  nu : Outport  Port=2
  deta : Outport  Port=3
  wires:
  Constant/1 -> MATLAB Function/5(del)
  Saturation2/1 -> Mux/6
  [nu] -> nu/1
  [eta] -> MATLAB Function1/1(eta)
  [eta] -> eta/1
  [eta] -> MATLAB Function/2(eta)
  [nu] -> MATLAB Function/1(nu)
  [nu] -> MATLAB Function1/2(nv)
  Saturation1/1 -> Mux/4
  MATLAB Function/1(dnu) -> Integrator/1
  tau_p/1 -> Subsystem/1(In1)
  Integrator1/1 -> Demux/1
  Integrator/1 -> [nu]
  MATLAB Function1/1(deta) -> Integrator1/1, deta/1
  tau_d/1 -> MATLAB Function/4(tau_d)
  Demux/1 -> Mux/1
  Demux/2 -> Mux/2
  Demux/3 -> Mux/3
  Demux/4 -> Saturation1/1
  Demux/5 -> Saturation/1
  Demux/6 -> Saturation2/1
  Mux/1 -> [eta]
  Saturation/1 -> Mux/5
  Subsystem/1(Out1) -> MATLAB Function/3(tau_p)

== system model/ADRC/控制器 ==
  r : Inport
  eta : Inport  Port=2
  dr : Inport  Port=3
  ddr : Inport  Port=4
  6路levant微分器 : Subsystem
  Constant : Constant  Value=wo
  MATLAB Function : MATLAB Function  TreatAsAtomicUnit=on
  Subsystem : Subsystem
  Subsystem1 : Subsystem
  Subsystem2 : Subsystem
  tau_p : Outport
  wires:
  MATLAB Function/2(u0) -> Subsystem1/1(tau_p)
  Subsystem1/2(x2) -> MATLAB Function/5(x2)
  Subsystem1/1(x1) -> MATLAB Function/4(x1)
  Subsystem1/3(x3) -> MATLAB Function/6(x3)
  eta/1 -> Subsystem1/3(eta), MATLAB Function/8(eta)
  ddr/1 -> MATLAB Function/3(ddr)
  dr/1 -> MATLAB Function/2(dr)
  Constant/1 -> MATLAB Function/7(wo)
  r/1 -> MATLAB Function/1(r)
  MATLAB Function/1(tau_p) -> Subsystem2/1(In1)
  Subsystem2/1(Out1) -> tau_p/1

== system model/FO_SMC/Subsystem ==
  y : Inport
  Demux : Demux  Outputs=6
  Mux : Mux  Inputs=6
  Mux1 : Mux  Inputs=6
  Mux2 : Mux  Inputs=6
  Subsystem1 : Subsystem  mask{a1=a1, a2=a2, a3=a3, a4=a4}
      mask DialogControl ParameterGroupVar Prompt: 参数
  Subsystem2 : Subsystem  mask{a1=a1, a2=a2, a3=a3, a4=a4}
      mask DialogControl ParameterGroupVar Prompt: 参数
  Subsystem3 : Subsystem  mask{a1=a1, a2=a2, a3=a3, a4=a4}
      mask DialogControl ParameterGroupVar Prompt: 参数
  Subsystem4 : Subsystem  mask{a1=a1, a2=a2, a3=a3, a4=a4}
      mask DialogControl ParameterGroupVar Prompt: 参数
  Subsystem5 : Subsystem  mask{a1=a1, a2=a2, a3=a3, a4=a4}
      mask DialogControl ParameterGroupVar Prompt: 参数
  Subsystem6 : Subsystem  mask{a1=a1, a2=a2, a3=a3, a4=a4}
      mask DialogControl ParameterGroupVar Prompt: 参数
  y_hat : Outport
  y1_hat : Outport  Port=2
  y1_hat1 : Outport  Port=3
  wires:
  Subsystem1/1(y_hat) -> Mux/2
  Demux/1 -> Subsystem4/1(y)
  Subsystem1/3(y1_hat1) -> Mux2/2
  Demux/2 -> Subsystem1/1(y)
  Subsystem4/1(y_hat) -> Mux/1
  Subsystem4/3(y1_hat1) -> Mux2/1
  y/1 -> Demux/1
  Mux/1 -> y_hat/1
  Demux/3 -> Subsystem2/1(y)
  Subsystem2/1(y_hat) -> Mux/3
  Demux/4 -> Subsystem3/1(y)
  Subsystem3/1(y_hat) -> Mux/4
  Demux/5 -> Subsystem5/1(y)
  Subsystem5/1(y_hat) -> Mux/5
  Demux/6 -> Subsystem6/1(y)
  Subsystem6/1(y_hat) -> Mux/6
  Subsystem6/2(y1_hat) -> Mux1/6
  Mux1/1 -> y1_hat/1
  Subsystem5/2(y1_hat) -> Mux1/5
  Subsystem3/2(y1_hat) -> Mux1/4
  Subsystem2/2(y1_hat) -> Mux1/3
  Subsystem1/2(y1_hat) -> Mux1/2
  Subsystem4/2(y1_hat) -> Mux1/1
  Subsystem2/3(y1_hat1) -> Mux2/3
  Subsystem3/3(y1_hat1) -> Mux2/4
  Subsystem5/3(y1_hat1) -> Mux2/5
  Subsystem6/3(y1_hat1) -> Mux2/6
  Mux2/1 -> y1_hat1/1

== system model/FO_SMC/Subsystem2 ==
  eta : Inport
  eta_d : Inport  Port=2
  MATLAB Function6 : MATLAB Function  TreatAsAtomicUnit=on
  Subsystem1 : Subsystem
  Out1 : Outport
  Out2 : Outport  Port=2
  wires:
  MATLAB Function6/1(e) -> Subsystem1/1(In1)
  eta_d/1 -> MATLAB Function6/2(x_d)
  Subsystem1/1(Out1) -> Out1/1
  eta/1 -> MATLAB Function6/1(x)
  Subsystem1/2(Out2) -> Out2/1

== system model/FO_SMC_ESO/LESO ==
  eta : Inport
  M_eta : Inport  Port=2
  J : Inport  Port=3
  J_inv : Inport  Port=4
  tau_c : Inport  Port=5
  MATLAB Function3 : MATLAB Function  TreatAsAtomicUnit=on
  MATLAB Function4 : MATLAB Function  TreatAsAtomicUnit=on
  Subsystem1 : Subsystem
  tau_2 : Outport
  h3 : Outport  Port=2
  wires:
  Subsystem1/1(tau_1) -> h3/1, MATLAB Function4/3(h3)
  tau_c/1 -> MATLAB Function3/3(tau_c)
  J_inv/1 -> MATLAB Function3/2(J_inv)
  M_eta/1 -> MATLAB Function4/2(M_eta), MATLAB Function3/1(M_eta)
  MATLAB Function3/1(tau_0) -> Subsystem1/2(In2)
  eta/1 -> Subsystem1/1(eta)
  J/1 -> MATLAB Function4/1(J)
  MATLAB Function4/1(tau_2) -> tau_2/1

== system model/FO_SMC_ESO/Levant微分器 ==
  y : Inport
  Demux : Demux  Outputs=6
  Mux : Mux  Inputs=6
  Mux1 : Mux  Inputs=6
  Mux2 : Mux  Inputs=6
  Subsystem1 : Subsystem  mask{a1=a1, a2=a2, a3=a3, a4=a4}
      mask DialogControl ParameterGroupVar Prompt: 参数
  Subsystem2 : Subsystem  mask{a1=a1, a2=a2, a3=a3, a4=a4}
      mask DialogControl ParameterGroupVar Prompt: 参数
  Subsystem3 : Subsystem  mask{a1=a1, a2=a2, a3=a3, a4=a4}
      mask DialogControl ParameterGroupVar Prompt: 参数
  Subsystem4 : Subsystem  mask{a1=a1, a2=a2, a3=a3, a4=a4}
      mask DialogControl ParameterGroupVar Prompt: 参数
  Subsystem5 : Subsystem  mask{a1=a1, a2=a2, a3=a3, a4=a4}
      mask DialogControl ParameterGroupVar Prompt: 参数
  Subsystem6 : Subsystem  mask{a1=a1, a2=a2, a3=a3, a4=a4}
      mask DialogControl ParameterGroupVar Prompt: 参数
  y_hat : Outport  PortDimensions=6
  y1_hat : Outport  Port=2
  y1_hat1 : Outport  Port=3
  wires:
  Subsystem1/1(y_hat) -> Mux/2
  Demux/1 -> Subsystem4/1(y)
  Subsystem1/3(y1_hat1) -> Mux2/2
  Demux/2 -> Subsystem1/1(y)
  Subsystem4/1(y_hat) -> Mux/1
  Subsystem4/3(y1_hat1) -> Mux2/1
  y/1 -> Demux/1
  Mux/1 -> y_hat/1
  Demux/3 -> Subsystem2/1(y)
  Subsystem2/1(y_hat) -> Mux/3
  Demux/4 -> Subsystem3/1(y)
  Subsystem3/1(y_hat) -> Mux/4
  Demux/5 -> Subsystem5/1(y)
  Subsystem5/1(y_hat) -> Mux/5
  Demux/6 -> Subsystem6/1(y)
  Subsystem6/1(y_hat) -> Mux/6
  Subsystem6/2(y1_hat) -> Mux1/6
  Mux1/1 -> y1_hat/1
  Subsystem5/2(y1_hat) -> Mux1/5
  Subsystem3/2(y1_hat) -> Mux1/4
  Subsystem2/2(y1_hat) -> Mux1/3
  Subsystem1/2(y1_hat) -> Mux1/2
  Subsystem4/2(y1_hat) -> Mux1/1
  Subsystem2/3(y1_hat1) -> Mux2/3
  Subsystem3/3(y1_hat1) -> Mux2/4
  Subsystem5/3(y1_hat1) -> Mux2/5
  Subsystem6/3(y1_hat1) -> Mux2/6
  Mux2/1 -> y1_hat1/1

== system model/FO_SMC_ESO/Subsystem1 ==
  y : Inport
  Demux : Demux  Outputs=6
  Mux : Mux  Inputs=6
  Out1 : Outport
  wires:
  Mux/1 -> Out1/1
  Demux/6 -> Mux/6
  Demux/5 -> Mux/5
  Demux/2 -> Mux/2
  Demux/1 -> Mux/1
  Demux/3 -> Mux/3
  y/1 -> Demux/1
  Demux/4 -> Mux/4

== system model/FO_SMC_ESO/Subsystem2 ==
  eta : Inport
  deta : Inport  Port=2
  eta1 : Inport  Port=3
  deta1 : Inport  Port=4
  MATLAB Function1 : MATLAB Function  TreatAsAtomicUnit=on
  线性反馈 : MATLAB Function  TreatAsAtomicUnit=on
  tau_1 : Outport
  M_eta : Outport  Port=2
  J : Outport  Port=3
  J_inv : Outport  Port=4
  wires:
  deta1/1 -> MATLAB Function1/2(deta)
  线性反馈/2(M_eta) -> M_eta/1
  MATLAB Function1/1(nu) -> 线性反馈/3(nu)
  线性反馈/3(J) -> J/1
  deta/1 -> 线性反馈/2(deta)
  线性反馈/4(J_inv) -> J_inv/1
  eta1/1 -> MATLAB Function1/1(eta)
  线性反馈/1(tau_1) -> tau_1/1
  eta/1 -> 线性反馈/1(eta)

== system model/FO_SMC_ESO/Subsystem3 ==
  eta : Inport
  eta1 : Inport  Port=2
  M_eta : Inport  Port=3
  J : Inport  Port=4
  deta : Inport  Port=5
  eta_d : Inport  Port=6
  deta_d : Inport  Port=7
  ddeta_d : Inport  Port=8
  h3 : Inport  Port=9
  Constant : Constant  Value=c1
  Constant1 : Constant  Value=c2
  Constant2 : Constant  Value=k
  Constant3 : Constant  Value=epsilon
  Delay : Delay  DelayLength=1  InitialCondition=[0;0;0;0;0;0]
  Subsystem2 : Subsystem
  分数阶滑模 : MATLAB Function  TreatAsAtomicUnit=on
  tau_3 : Outport
  wires:
  ddeta_d/1 -> 分数阶滑模/9(ddeta_d)
  Subsystem2/2(D2) -> 分数阶滑模/4(D2)
  deta_d/1 -> 分数阶滑模/8(deta_d)
  Constant2/1 -> 分数阶滑模/10(k0)
  eta_d/1 -> Subsystem2/2(eta_d), 分数阶滑模/7(eta_d)
  Constant3/1 -> 分数阶滑模/11(epsilon0)
  Subsystem2/1(D1) -> 分数阶滑模/3(D1)
  Constant1/1 -> 分数阶滑模/6(c2)
  Constant/1 -> 分数阶滑模/5(c1)
  J/1 -> 分数阶滑模/12(J)
  M_eta/1 -> 分数阶滑模/13(M_eta)
  分数阶滑模/1(tau_3) -> tau_3/1
  eta1/1 -> Subsystem2/1(eta)
  deta/1 -> 分数阶滑模/2(deta)
  eta/1 -> 分数阶滑模/1(eta)
  分数阶滑模/2(ds) -> Delay/1
  h3/1 -> 分数阶滑模/14(h3)
  Delay/1 -> ?

== system model/FO_SMC_T/Subsystem ==
  y : Inport
  Demux : Demux  Outputs=6
  Mux : Mux  Inputs=6
  Mux1 : Mux  Inputs=6
  Mux2 : Mux  Inputs=6
  Subsystem1 : Subsystem  mask{a1=a1, a2=a2, a3=a3, a4=a4}
      mask DialogControl ParameterGroupVar Prompt: 参数
  Subsystem2 : Subsystem  mask{a1=a1, a2=a2, a3=a3, a4=a4}
      mask DialogControl ParameterGroupVar Prompt: 参数
  Subsystem3 : Subsystem  mask{a1=a1, a2=a2, a3=a3, a4=a4}
      mask DialogControl ParameterGroupVar Prompt: 参数
  Subsystem4 : Subsystem  mask{a1=a1, a2=a2, a3=a3, a4=a4}
      mask DialogControl ParameterGroupVar Prompt: 参数
  Subsystem5 : Subsystem  mask{a1=a1, a2=a2, a3=a3, a4=a4}
      mask DialogControl ParameterGroupVar Prompt: 参数
  Subsystem6 : Subsystem  mask{a1=a1, a2=a2, a3=a3, a4=a4}
      mask DialogControl ParameterGroupVar Prompt: 参数
  y_hat : Outport
  y1_hat : Outport  Port=2
  y1_hat1 : Outport  Port=3
  wires:
  Subsystem1/1(y_hat) -> Mux/2
  Demux/1 -> Subsystem4/1(y)
  Subsystem1/3(y1_hat1) -> Mux2/2
  Demux/2 -> Subsystem1/1(y)
  Subsystem4/1(y_hat) -> Mux/1
  Subsystem4/3(y1_hat1) -> Mux2/1
  y/1 -> Demux/1
  Mux/1 -> y_hat/1
  Demux/3 -> Subsystem2/1(y)
  Subsystem2/1(y_hat) -> Mux/3
  Demux/4 -> Subsystem3/1(y)
  Subsystem3/1(y_hat) -> Mux/4
  Demux/5 -> Subsystem5/1(y)
  Subsystem5/1(y_hat) -> Mux/5
  Demux/6 -> Subsystem6/1(y)
  Subsystem6/1(y_hat) -> Mux/6
  Subsystem6/2(y1_hat) -> Mux1/6
  Mux1/1 -> y1_hat/1
  Subsystem5/2(y1_hat) -> Mux1/5
  Subsystem3/2(y1_hat) -> Mux1/4
  Subsystem2/2(y1_hat) -> Mux1/3
  Subsystem1/2(y1_hat) -> Mux1/2
  Subsystem4/2(y1_hat) -> Mux1/1
  Subsystem2/3(y1_hat1) -> Mux2/3
  Subsystem3/3(y1_hat1) -> Mux2/4
  Subsystem5/3(y1_hat1) -> Mux2/5
  Subsystem6/3(y1_hat1) -> Mux2/6
  Mux2/1 -> y1_hat1/1

== system model/FO_SMC_T/Subsystem2 ==
  eta : Inport
  eta_d : Inport  Port=2
  MATLAB Function6 : MATLAB Function  TreatAsAtomicUnit=on
  Subsystem1 : Subsystem
  Out1 : Outport
  Out2 : Outport  Port=2
  wires:
  MATLAB Function6/1(e) -> Subsystem1/1(In1)
  eta_d/1 -> MATLAB Function6/2(x_d)
  Subsystem1/1(Out1) -> Out1/1
  eta/1 -> MATLAB Function6/1(x)
  Subsystem1/2(Out2) -> Out2/1

== system model/SMC/Subsystem ==
  y : Inport
  Demux : Demux  Outputs=6
  Mux : Mux  Inputs=6
  Mux1 : Mux  Inputs=6
  Mux2 : Mux  Inputs=6
  Subsystem1 : Subsystem  mask{a1=a1, a2=a2, a3=a3, a4=a4}
      mask DialogControl ParameterGroupVar Prompt: 参数
  Subsystem2 : Subsystem  mask{a1=a1, a2=a2, a3=a3, a4=a4}
      mask DialogControl ParameterGroupVar Prompt: 参数
  Subsystem3 : Subsystem  mask{a1=a1, a2=a2, a3=a3, a4=a4}
      mask DialogControl ParameterGroupVar Prompt: 参数
  Subsystem4 : Subsystem  mask{a1=a1, a2=a2, a3=a3, a4=a4}
      mask DialogControl ParameterGroupVar Prompt: 参数
  Subsystem5 : Subsystem  mask{a1=a1, a2=a2, a3=a3, a4=a4}
      mask DialogControl ParameterGroupVar Prompt: 参数
  Subsystem6 : Subsystem  mask{a1=a1, a2=a2, a3=a3, a4=a4}
      mask DialogControl ParameterGroupVar Prompt: 参数
  y_hat : Outport
  y1_hat : Outport  Port=2
  y1_hat1 : Outport  Port=3
  wires:
  Subsystem1/1(y_hat) -> Mux/2
  Demux/1 -> Subsystem4/1(y)
  Subsystem1/3(y1_hat1) -> Mux2/2
  Demux/2 -> Subsystem1/1(y)
  Subsystem4/1(y_hat) -> Mux/1
  Subsystem4/3(y1_hat1) -> Mux2/1
  y/1 -> Demux/1
  Mux/1 -> y_hat/1
  Demux/3 -> Subsystem2/1(y)
  Subsystem2/1(y_hat) -> Mux/3
  Demux/4 -> Subsystem3/1(y)
  Subsystem3/1(y_hat) -> Mux/4
  Demux/5 -> Subsystem5/1(y)
  Subsystem5/1(y_hat) -> Mux/5
  Demux/6 -> Subsystem6/1(y)
  Subsystem6/1(y_hat) -> Mux/6
  Subsystem6/2(y1_hat) -> Mux1/6
  Mux1/1 -> y1_hat/1
  Subsystem5/2(y1_hat) -> Mux1/5
  Subsystem3/2(y1_hat) -> Mux1/4
  Subsystem2/2(y1_hat) -> Mux1/3
  Subsystem1/2(y1_hat) -> Mux1/2
  Subsystem4/2(y1_hat) -> Mux1/1
  Subsystem2/3(y1_hat1) -> Mux2/3
  Subsystem3/3(y1_hat1) -> Mux2/4
  Subsystem5/3(y1_hat1) -> Mux2/5
  Subsystem6/3(y1_hat1) -> Mux2/6
  Mux2/1 -> y1_hat1/1

== system model/系统1/Subsystem ==
  In1 : Inport
  Demux1 : Demux  Outputs=6
  Mux1 : Mux  Inputs=6
  Saturation{1..6} (6 alike) : Saturate  UpperLimit=tau_p_max  LowerLimit=-tau_p_max
  Out1 : Outport
  wires:
  Saturation6/1 -> Mux1/6
  Saturation3/1 -> Mux1/3
  Saturation2/1 -> Mux1/2
  Saturation1/1 -> Mux1/1
  Mux1/1 -> Out1/1
  In1/1 -> Demux1/1
  Demux1/4 -> Saturation4/1
  Demux1/6 -> Saturation6/1
  Demux1/1 -> Saturation1/1
  Demux1/5 -> Saturation5/1
  Saturation5/1 -> Mux1/5
  Demux1/3 -> Saturation3/1
  Saturation4/1 -> Mux1/4
  Demux1/2 -> Saturation2/1

== system model/系统2/Subsystem ==
  In1 : Inport
  Demux1 : Demux  Outputs=6
  Mux1 : Mux  Inputs=6
  Saturation{1..6} (6 alike) : Saturate  UpperLimit=tau_p_max  LowerLimit=-tau_p_max
  Out1 : Outport
  wires:
  Demux1/2 -> Saturation2/1
  Saturation4/1 -> Mux1/4
  Demux1/3 -> Saturation3/1
  Saturation5/1 -> Mux1/5
  Demux1/5 -> Saturation5/1
  Demux1/1 -> Saturation1/1
  Demux1/6 -> Saturation6/1
  Demux1/4 -> Saturation4/1
  In1/1 -> Demux1/1
  Mux1/1 -> Out1/1
  Saturation1/1 -> Mux1/1
  Saturation2/1 -> Mux1/2
  Saturation3/1 -> Mux1/3
  Saturation6/1 -> Mux1/6

== system model/系统3/Subsystem ==
  In1 : Inport
  Demux1 : Demux  Outputs=6
  Mux1 : Mux  Inputs=6
  Saturation{1..6} (6 alike) : Saturate  UpperLimit=tau_p_max  LowerLimit=-tau_p_max
  Out1 : Outport
  wires:
  Saturation6/1 -> Mux1/6
  Saturation3/1 -> Mux1/3
  Saturation2/1 -> Mux1/2
  Saturation1/1 -> Mux1/1
  Mux1/1 -> Out1/1
  In1/1 -> Demux1/1
  Demux1/4 -> Saturation4/1
  Demux1/6 -> Saturation6/1
  Demux1/1 -> Saturation1/1
  Demux1/5 -> Saturation5/1
  Saturation5/1 -> Mux1/5
  Demux1/3 -> Saturation3/1
  Saturation4/1 -> Mux1/4
  Demux1/2 -> Saturation2/1

== system model/系统4/Subsystem ==
  In1 : Inport
  Demux1 : Demux  Outputs=6
  Mux1 : Mux  Inputs=6
  Saturation{1..6} (6 alike) : Saturate  UpperLimit=tau_p_max  LowerLimit=-tau_p_max
  Out1 : Outport
  wires:
  Demux1/2 -> Saturation2/1
  Saturation4/1 -> Mux1/4
  Demux1/3 -> Saturation3/1
  Saturation5/1 -> Mux1/5
  Demux1/5 -> Saturation5/1
  Demux1/1 -> Saturation1/1
  Demux1/6 -> Saturation6/1
  Demux1/4 -> Saturation4/1
  In1/1 -> Demux1/1
  Mux1/1 -> Out1/1
  Saturation1/1 -> Mux1/1
  Saturation2/1 -> Mux1/2
  Saturation3/1 -> Mux1/3
  Saturation6/1 -> Mux1/6

== system model/系统5/Subsystem ==
  In1 : Inport
  Demux1 : Demux  Outputs=6
  Mux1 : Mux  Inputs=6
  Saturation{1..6} (6 alike) : Saturate  UpperLimit=tau_p_max  LowerLimit=-tau_p_max
  Out1 : Outport
  wires:
  Demux1/2 -> Saturation2/1
  Saturation4/1 -> Mux1/4
  Demux1/3 -> Saturation3/1
  Saturation5/1 -> Mux1/5
  Demux1/5 -> Saturation5/1
  Demux1/1 -> Saturation1/1
  Demux1/6 -> Saturation6/1
  Demux1/4 -> Saturation4/1
  In1/1 -> Demux1/1
  Mux1/1 -> Out1/1
  Saturation1/1 -> Mux1/1
  Saturation2/1 -> Mux1/2
  Saturation3/1 -> Mux1/3
  Saturation6/1 -> Mux1/6

== system model/ADRC/控制器/6路levant微分器 ==
  y : Inport
  Demux : Demux  Outputs=6
  Mux : Mux  Inputs=6
  Mux1 : Mux  Inputs=6
  Mux2 : Mux  Inputs=6
  Subsystem1 : Subsystem
  Subsystem2 : Subsystem
  Subsystem3 : Subsystem
  Subsystem4 : Subsystem
  Subsystem5 : Subsystem
  Subsystem6 : Subsystem
  y_hat : Outport
  dy_hat : Outport  Port=2
  ddy_hat : Outport  Port=3
  wires:
  Mux2/1 -> ddy_hat/1
  Subsystem6/3(y1_hat1) -> Mux2/6
  Subsystem5/3(y1_hat1) -> Mux2/5
  Subsystem3/3(y1_hat1) -> Mux2/4
  Subsystem2/3(y1_hat1) -> Mux2/3
  Subsystem4/2(y1_hat) -> Mux1/1
  Subsystem1/2(y1_hat) -> Mux1/2
  Subsystem2/2(y1_hat) -> Mux1/3
  Subsystem3/2(y1_hat) -> Mux1/4
  Subsystem5/2(y1_hat) -> Mux1/5
  Mux1/1 -> dy_hat/1
  Subsystem6/2(y1_hat) -> Mux1/6
  Subsystem6/1(y_hat) -> Mux/6
  Demux/6 -> Subsystem6/1(y)
  Subsystem5/1(y_hat) -> Mux/5
  Demux/5 -> Subsystem5/1(y)
  Subsystem3/1(y_hat) -> Mux/4
  Demux/4 -> Subsystem3/1(y)
  Subsystem2/1(y_hat) -> Mux/3
  Demux/3 -> Subsystem2/1(y)
  Mux/1 -> y_hat/1
  y/1 -> Demux/1
  Subsystem4/3(y1_hat1) -> Mux2/1
  Subsystem4/1(y_hat) -> Mux/1
  Demux/2 -> Subsystem1/1(y)
  Subsystem1/3(y1_hat1) -> Mux2/2
  Demux/1 -> Subsystem4/1(y)
  Subsystem1/1(y_hat) -> Mux/2

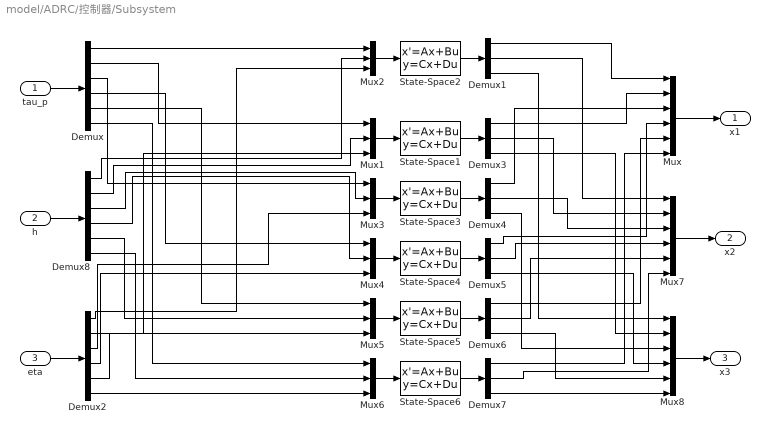
== system model/ADRC/控制器/Subsystem ==
  tau_p : Inport
  h : Inport  Port=2
  eta : Inport  Port=3
  Demux : Demux  Outputs=6
  Demux{1,3..7} (6 alike) : Demux  Outputs=3
  Demux2 : Demux  Outputs=6
  Demux8 : Demux  Outputs=6
  Mux : Mux  Inputs=6
  Mux{1..6} (6 alike) : Mux  Inputs=3
  Mux7 : Mux  Inputs=6
  Mux8 : Mux  Inputs=6
  State-Space{1..6} (6 alike) : StateSpace  A=[-3*w 1 0;-3*w^2 0 1;-w^3 0 0]  B=[0 0 3*w;1 0 3*w^2;0 1 w^3]  C=[1 0 0;0 1 0;0 0 1]  D=[0 0 0;0 0 0;0 0 0]  InitialCondition=0
  x1 : Outport
  x2 : Outport  Port=2
  x3 : Outport  Port=3
  wires:
  h/1 -> Demux8/1
  Demux7/3 -> Mux8/6
  Demux6/3 -> Mux8/5
  Demux5/3 -> Mux8/4
  Demux4/3 -> Mux8/3
  Demux3/3 -> Mux8/2
  Mux8/1 -> x3/1
  Demux1/3 -> Mux8/1
  Demux1/2 -> Mux7/1
  Mux7/1 -> x2/1
  Demux3/2 -> Mux7/2
  Demux4/2 -> Mux7/3
  Demux5/2 -> Mux7/4
  Demux6/2 -> Mux7/5
  Demux7/2 -> Mux7/6
  Demux/6 -> Mux6/1
  Demux/5 -> Mux5/1
  Demux/4 -> Mux4/1
  Demux/3 -> Mux3/1
  State-Space6/1 -> Demux7/1
  Mux6/1 -> State-Space6/1
  Demux2/6 -> Mux6/3
  Demux7/1 -> Mux/6
  Demux8/6 -> Mux6/2
  Demux8/5 -> Mux5/2
  Demux6/1 -> Mux/5
  Demux2/5 -> Mux5/3
  Mux5/1 -> State-Space5/1
  State-Space5/1 -> Demux6/1
  State-Space4/1 -> Demux5/1
  Mux4/1 -> State-Space4/1
  Demux2/4 -> Mux4/3
  Demux5/1 -> Mux/4
  Demux8/4 -> Mux4/2
  Demux8/3 -> Mux3/2
  Demux4/1 -> Mux/3
  Demux2/3 -> Mux3/3
  Mux3/1 -> State-Space3/1
  State-Space3/1 -> Demux4/1
  State-Space1/1 -> Demux3/1
  Mux1/1 -> State-Space1/1
  Demux/2 -> Mux1/1
  Demux2/2 -> Mux1/3
  Demux3/1 -> Mux/2
  Demux8/2 -> Mux1/2
  Mux/1 -> x1/1
  eta/1 -> Demux2/1
  tau_p/1 -> Demux/1
  Demux8/1 -> Mux2/2
  Demux1/1 -> Mux/1
  Demux2/1 -> Mux2/3
  Demux/1 -> Mux2/1
  Mux2/1 -> State-Space2/1
  State-Space2/1 -> Demux1/1

== system model/ADRC/控制器/Subsystem1 ==
  tau_p : Inport
  h : Inport  Port=2
  eta : Inport  Port=3
  Demux : Demux  Outputs=6
  Demux2 : Demux  Outputs=6
  Demux8 : Demux  Outputs=6
  Mux : Mux  Inputs=6
  Mux7 : Mux  Inputs=6
  Mux8 : Mux  Inputs=6
  Subsystem1 : Subsystem
  Subsystem2 : Subsystem
  Subsystem3 : Subsystem
  Subsystem4 : Subsystem
  Subsystem5 : Subsystem
  Subsystem6 : Subsystem
  x1 : Outport
  x2 : Outport  Port=2
  x3 : Outport  Port=3
  wires:
  tau_p/1 -> Demux/1
  eta/1 -> Demux2/1
  Mux/1 -> x1/1
  Mux7/1 -> x2/1
  Mux8/1 -> x3/1
  h/1 -> Demux8/1
  Demux/1 -> Subsystem6/1(tau_0)
  Demux2/1 -> Subsystem6/2(eta)
  Subsystem6/1(Out3) -> Mux/1
  Subsystem6/2(Out1) -> Mux7/1
  Subsystem6/3(Out2) -> Mux8/1
  Demux2/2 -> Subsystem1/2(eta)
  Subsystem1/1(Out3) -> Mux/2
  Subsystem1/2(Out1) -> Mux7/2
  Subsystem1/3(Out2) -> Mux8/2
  Subsystem2/3(Out2) -> Mux8/3
  Subsystem2/2(Out1) -> Mux7/3
  Subsystem2/1(Out3) -> Mux/3
  Demux2/3 -> Subsystem2/2(eta)
  Demux/2 -> Subsystem1/1(tau_0)
  Demux/3 -> Subsystem2/1(tau_0)
  Demux/4 -> Subsystem3/1(tau_0)
  Demux2/4 -> Subsystem3/2(eta)
  Subsystem3/1(Out3) -> Mux/4
  Subsystem3/3(Out2) -> Mux8/4
  Subsystem3/2(Out1) -> Mux7/4
  Demux/5 -> Subsystem4/1(tau_0)
  Demux2/5 -> Subsystem4/2(eta)
  Subsystem4/1(Out3) -> Mux/5
  Subsystem4/2(Out1) -> Mux7/5
  Subsystem4/3(Out2) -> Mux8/5
  Demux/6 -> Subsystem5/1(tau_0)
  Demux2/6 -> Subsystem5/2(eta)
  Subsystem5/1(Out3) -> Mux/6
  Subsystem5/2(Out1) -> Mux7/6
  Subsystem5/3(Out2) -> Mux8/6

== system model/ADRC/控制器/Subsystem2 ==
  In1 : Inport
  Demux : Demux  Outputs=6
  Mux : Mux  Inputs=6
  Out1 : Outport
  wires:
  Mux/1 -> Out1/1
  Demux/6 -> Mux/6
  Demux/5 -> Mux/5
  Demux/2 -> Mux/2
  Demux/1 -> Mux/1
  Demux/3 -> Mux/3
  In1/1 -> Demux/1
  Demux/4 -> Mux/4
